simulink model "cont_modifed"  (Simulink 5.0)
settings: Solver=ode45  StartTime=0.0  StopTime=10.0  RelTol=1e-3
settings Model: LastModifiedBy=dev

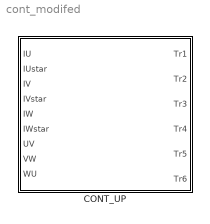
== system cont_modifed ==
  CONT_UP : Stateflow chart  TreatAsAtomicUnit=on

== stateflow chart CONT_UP ==
  settings: updateMethod=CONTINUOUS  sampleTime=0.0001
  state A/
    state A11/
      during:Tr1=0;Tr1=0;Tr2=0;Tr3=0;Tr4=0;Tr5=0;
      Tr6=0;
    state A2/
      during: Tr1=0; Tr3=0; Tr4=0; Tr2=0; Tr5=1;
      Tr6=0;
  state B/
    state B1/
      during: Tr3=0;Tr5=0;Tr4=0;Tr2=0;
      Tr1=0; Tr6=0;
    state B2/
      during:Tr3=0;Tr5=0;Tr4=0;Tr2=0;
      Tr1=1; Tr6=0;
    (default) -> B1
  state C/
    state C1/
      during: Tr3=0;Tr5=0;Tr4=0;Tr2=0;
      Tr1=0; Tr6=0;
    state C2/
      during: Tr3=0;Tr5=0; Tr4=0; Tr6=0;
      Tr1=1; Tr2=0;
    (default) -> C1
  state D/
    state D1/
      during: Tr3=0;Tr5=0;Tr4=0;Tr2=0;
      Tr1=0; Tr6=0;
    state D2/
      during: Tr1=0; Tr5=0;Tr4=0; Tr6=0;
      Tr3=1; Tr2=0;
    (default) -> D1
  state E/
    state E1/
      during: Tr3=0;Tr5=0;Tr4=0;Tr2=0;
      Tr1=0; Tr6=0;
    state E2/
      during: Tr1=0; Tr5=0; Tr6=0; Tr2=0;
      Tr3=1; Tr4=0;
    (default) -> E1
  state F/
    state F1/
      during: Tr3=0;Tr5=0;Tr4=0;Tr2=0;
      Tr1=0; Tr6=0;
    state F2/
      during: Tr1=0; Tr3=0; Tr6=0; Tr2=0;
      Tr5=1; Tr4=0;
    (default) -> F1
  (default) -> A : [1]
  A2 -> A11 : [IWstar<IW]
  B1 -> B2 : [IU <IUstar]
  B2 -> B1 : [IU>IUstar]
  A -> B : [WU==1]
  C1 -> C2 : [IUstar>IU]
  C2 -> C1 : [IUstar<IU]
  B -> C : [VW==1]
  D1 -> D2 : [IV<IVstar]
  D2 -> D1 : [IV>IVstar]
  C -> D : [UV==1]
  E1 -> E2 : [IVstar>IV]
  E2 -> E1 : [IVstar<IV]
  D -> E : [WU==1]
  F -> A : [UV==1]
  F1 -> F2 : [IW<IWstar]
  F2 -> F1 : [IW>IWstar]
  E -> F : [VW==1]
  A11 -> A2 : [IWstar>IW]
  data: IU input double; IUstar input double; IV input double; IVstar input double; IW input double; IWstar input double; Tr1 output double; Tr2 output double; Tr3 output double; Tr4 output double; Tr5 output double; Tr6 output double; UV input double; VW input double; WU input double
